simulink model "CBE_145_HW4_P2b"  (R2020b)
settings: Solver=VariableStepAuto  StartTime=0.0  StopTime=25  RelTol=1e-3
settings Model: SimulationMode=rapid-accelerator  Creator=Jesus Vergara  LastModifiedBy=Jesus Vergara

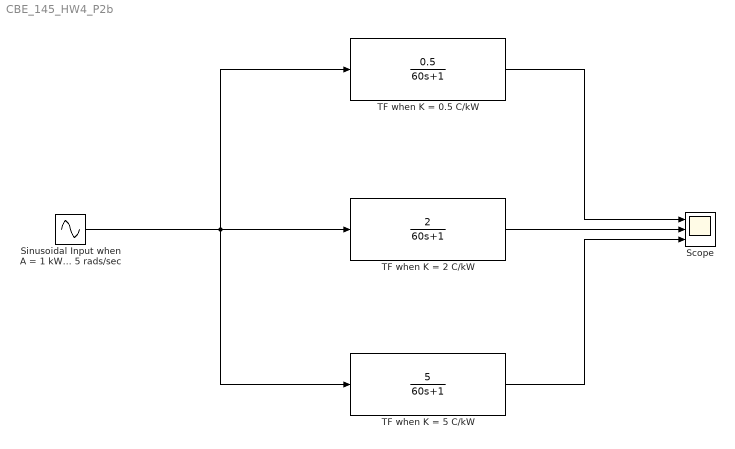
== system CBE_145_HW4_P2b ==
  Scope : Scope  NumInputPorts=3
  Sinusoidal Input when A = 1 kW and f = 5 rads/sec : Sin  Frequency=5  SampleTime=0
  TF when K = 0.5 C/kW : TransferFcn  Numerator=[0.5]  Denominator=[60 1]
  TF when K = 2 C/kW : TransferFcn  Numerator=[2]  Denominator=[60 1]
  TF when K = 5 C/kW : TransferFcn  Numerator=[5]  Denominator=[60 1]
  wires:
  TF when K = 0.5 C/kW/1 -> Scope/1
  TF when K = 5 C/kW/1 -> Scope/3
  Sinusoidal Input when A = 1 kW and f = 5 rads/sec/1 -> TF when K = 0.5 C/kW/1, TF when K = 5 C/kW/1, TF when K = 2 C/kW/1
  TF when K = 2 C/kW/1 -> Scope/2
